simulink model "PV_math_single_solar_cell"  (R2022a)
settings: Solver=VariableStepAuto  StartTime=0.0  StopTime=10.0  RelTol=1e-3
libraries: simulink x1
settings Model: Creator=Home computer  LastModifiedBy=Home computer

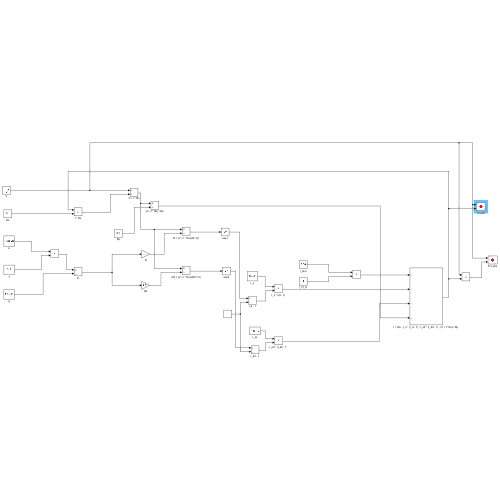
[thumbnail: Simulink's stored preview of the top-level diagram]
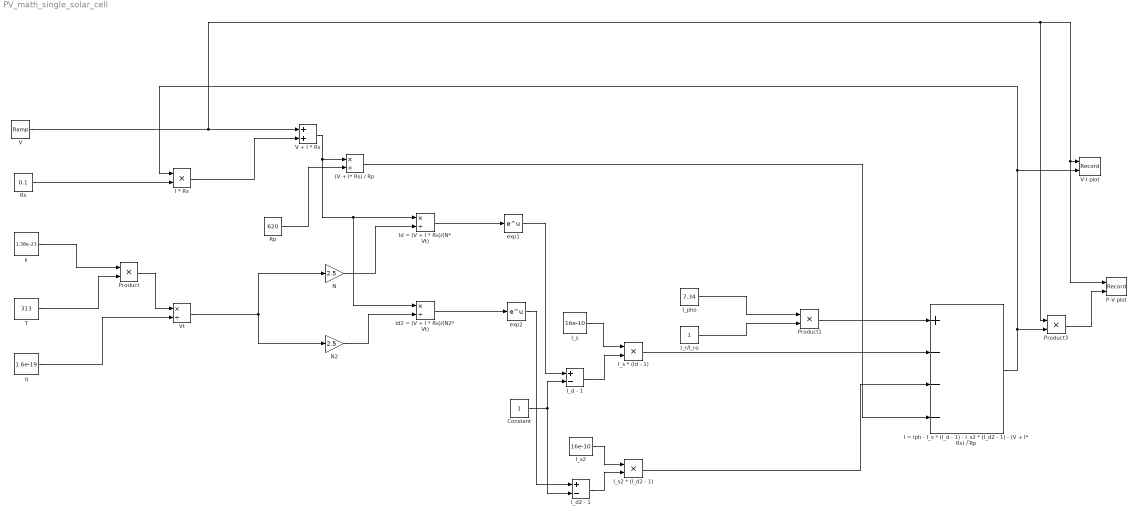
== system PV_math_single_solar_cell ==
  (V + I* Rs) / Rp : Product  Inputs=*/
  Constant : Constant
  I * Rs : Product
  "I = Iph - I_s * (I_d - 1) - I_s2 * (I_d2 - 1) - (V + I* Rs) / Rp " : Sum  Inputs=+---
  I_d - 1 : Sum  Inputs=+-
  I_d2 - 1 : Sum  Inputs=+-
  I_pho : Constant  Value=7.34
  I_r/I_ro : Constant
  I_s : Constant  Value=16e-10
  I_s * (Id - 1) : Product
  I_s2 : Constant  Value=16e-10
  I_s2 * (I_d2 - 1) : Product
  Id = (V + I * Rs)/(N* Vt) : Product  Inputs=*/
  Id2 = (V + I * Rs)/(N2* Vt) : Product  Inputs=*/
  N : Gain  Gain=2.5
  N2 : Gain  Gain=2.5
  P-V plot : Record  FileSettingsInternal="{\"entries\":[{\"content\":{\"excelSettings\":{\"content\":{},\"type\":\"Streamout.ExcelSettings\"}},\"type\":\"Streamout.FileSettingStorage\",\"uuid\":\"57035c88-3473-4834-ba80-ebb355cd837b\"}],\"packageUris\":[\"http://schema.mathworks.com/mf0/streamout_blocks/R2020a\"],\"version\":\"1.0\"}"  Layout=[1 1]  SignalsInternal="{\"entries\":[{\"content\":{\"signals\":[{\"content\":{\"blockPath\":[\"untitled/P-V plot\"],\"channel\":[],\"dimensions\":[1],\"domain\":\"untitled/P-V plot\",\"lineColor\":\"#a2142f\",\"plots\":[1],\"port\":1,\"sid\":[\"\"],\"signalID\":99,\"signalName\":\"V\"},\"type\":\"RecordBlkView.Signal\",\"uuid\":\"ea3e44e9-3b87-4695-9b39-1f09a10edc1b\"},{\"content\":{\"blockPath\":[\"untitled/P-V plot\"],\"channel\":[],\"dimensions\":[1],\"domain\":\"untitled/P-V plot\",\"lineColor\":\"#139fff\",\"plots\":[1],\"port\":2,\"sid\":[\"\"],\"signalID\":103,\"signalName\":\"Product3\"},\"type\":\"RecordBlkView.Signal\",\"uuid\":\"b0bd5d8d-11e6-46c3-915f-5139aee80ace\"}]},\"type\":\"RecordBlkView.InputSignals\",\"uuid\":\"70447eb7-407b-424a-a499-b51fa95d95e2\"}],\"packageUris\":[\"http://schema.mathworks.com/mf0/streamout_blocks/R2020a\"],\"version\":\"1.0\"}"  VisualizationBindings="{\"xyplotplugin\":{\"info\":[{\"series\":[{\"bindingParametersList\":[{\"parameter\":\"X-Axis\",\"signalID\":99,\"signalName\":\"V\"},{\"parameter\":\"Y-Axis\",\"signalID\":103,\"signalName\":\"Product3\"}],\"seriesID\":51317}],\"subplotID\":1}]}}"  CompatibilityTag=XY
  Product : Product
  Product1 : Product
  Product3 : Product
  Rp : Constant  Value=620
  Rs : Constant  Value=0.1
  T : Constant  Value=313
  V : simulink/Sources/Ramp  slope=1  start=0  InitialOutput=0
  V + I * Rs : Sum
  V-I plot : Record  FileSettingsInternal="{\"entries\":[{\"content\":{\"excelSettings\":{\"content\":{},\"type\":\"Streamout.ExcelSettings\"}},\"type\":\"Streamout.FileSettingStorage\",\"uuid\":\"5f0f6a2b-860a-4f32-99a7-6e79b1d32719\"}],\"packageUris\":[\"http://schema.mathworks.com/mf0/streamout_blocks/R2020a\"],\"version\":\"1.0\"}"  Layout=[1 1]  SignalsInternal="{\"entries\":[{\"content\":{\"signals\":[{\"content\":{\"blockPath\":[\"untitled/V-I plot\"],\"channel\":[],\"dimensions\":[1],\"domain\":\"untitled/V-I plot\",\"lineColor\":\"#a2142f\",\"plots\":[1],\"port\":1,\"sid\":[\"\"],\"signalID\":107,\"signalName\":\"V\"},\"type\":\"RecordBlkView.Signal\",\"uuid\":\"6513eb1b-8a24-42be-9406-77639d88ac99\"},{\"content\":{\"blockPath\":[\"untitled/V-I plot\"],\"channel\":[],\"dimensions\":[1],\"domain\":\"untitled/V-I plot\",\"lineColor\":\"#139fff\",\"plots\":[1],\"port\":2,\"sid\":[\"\"],\"signalID\":111,\"signalName\":\"I = Iph - I_s * (I_d - 1) - I_s2 * (I_d2 - 1) - (V + I* Rs) / Rp \"},\"type\":\"RecordBlkView.Signal\",\"uuid\":\"305aeb5c-741d-491a-87ad-55b5d7418bca\"}]},\"type\":\"RecordBlkView.InputSignals\",\"uuid\":\"9e631692-54c0-4563-b45e-8b79fefa61f2\"}],\"packageUris\":[\"http://schema.mathworks.com/mf0/streamout_blocks/R2020a\"],\"version\":\"1.0\"}"  VisualizationBindings="{\"xyplotplugin\":{\"info\":[{\"series\":[{\"bindingParametersList\":[{\"parameter\":\"X-Axis\",\"signalID\":107,\"signalName\":\"V\"},{\"parameter\":\"Y-Axis\",\"signalID\":111,\"signalName\":\"I = Iph - I_s * (I_d - 1) - I_s2 * (I_d2 - 1) - (V + I* Rs) \\/ Rp \"}],\"seriesID\":14225}],\"subplotID\":1}]}}"  CompatibilityTag=XY
  Vt : Product  Inputs=*/
  exp1 : Math
  exp2 : Math
  k : Constant  Value=1.38e-23
  q : Constant  Value=1.6e-19
  wires:
  k/1 -> Product/1
  T/1 -> Product/2
  Product/1 -> Vt/1
  q/1 -> Vt/2
  Rs/1 -> I * Rs/2
  V/1 -> Product3/1, P-V plot/1, V-I plot/1, V + I * Rs/1
  I * Rs/1 -> V + I * Rs/2
  V + I * Rs/1 -> (V + I* Rs) / Rp/1, Id2 = (V + I * Rs)/(N2* Vt)/1, Id = (V + I * Rs)/(N* Vt)/1
  Rp/1 -> (V + I* Rs) / Rp/2
  N/1 -> Id = (V + I * Rs)/(N* Vt)/2
  Vt/1 -> N2/1, N/1
  N2/1 -> Id2 = (V + I * Rs)/(N2* Vt)/2
  Id = (V + I * Rs)/(N* Vt)/1 -> exp1/1
  Id2 = (V + I * Rs)/(N2* Vt)/1 -> exp2/1
  exp1/1 -> I_d - 1/1
  Constant/1 -> I_d2 - 1/2, I_d - 1/2
  exp2/1 -> I_d2 - 1/1
  I_d - 1/1 -> I_s * (Id - 1)/2
  I_s/1 -> I_s * (Id - 1)/1
  I_s2/1 -> I_s2 * (I_d2 - 1)/1
  I_d2 - 1/1 -> I_s2 * (I_d2 - 1)/2
  I_r/I_ro/1 -> Product1/2
  I_pho/1 -> Product1/1
  Product1/1 -> "I = Iph - I_s * (I_d - 1) - I_s2 * (I_d2 - 1) - (V + I* Rs) / Rp "/1
  I_s * (Id - 1)/1 -> "I = Iph - I_s * (I_d - 1) - I_s2 * (I_d2 - 1) - (V + I* Rs) / Rp "/2
  I_s2 * (I_d2 - 1)/1 -> "I = Iph - I_s * (I_d - 1) - I_s2 * (I_d2 - 1) - (V + I* Rs) / Rp "/3
  (V + I* Rs) / Rp/1 -> "I = Iph - I_s * (I_d - 1) - I_s2 * (I_d2 - 1) - (V + I* Rs) / Rp "/4
  "I = Iph - I_s * (I_d - 1) - I_s2 * (I_d2 - 1) - (V + I* Rs) / Rp "/1 -> Product3/2, V-I plot/2, I * Rs/1
  Product3/1 -> P-V plot/2
